simulink model "prs_agc"  (Simulink 8.7)
settings: Solver=ode45  StartTime=0.0  StopTime=100  RelTol=1e-3
values from neighbouring files (symbols this model uses):
  kd = GlobalBest.Position(3)    [prs_PSO.m]
  ki = GlobalBest.Position(2)    [prs_PSO.m]
  kp = GlobalBest.Position(1)    [prs_PSO.m]
libraries: simulink x2
settings Model: Creator=Prasun-EE  LastModifiedBy=User
settings DebuggingCC: UnderspecifiedInitializationDetection=Simplified  MergeDetectMultiDrivingBlocksExec=error
settings ConfigComp: CovSFcnEnable=off

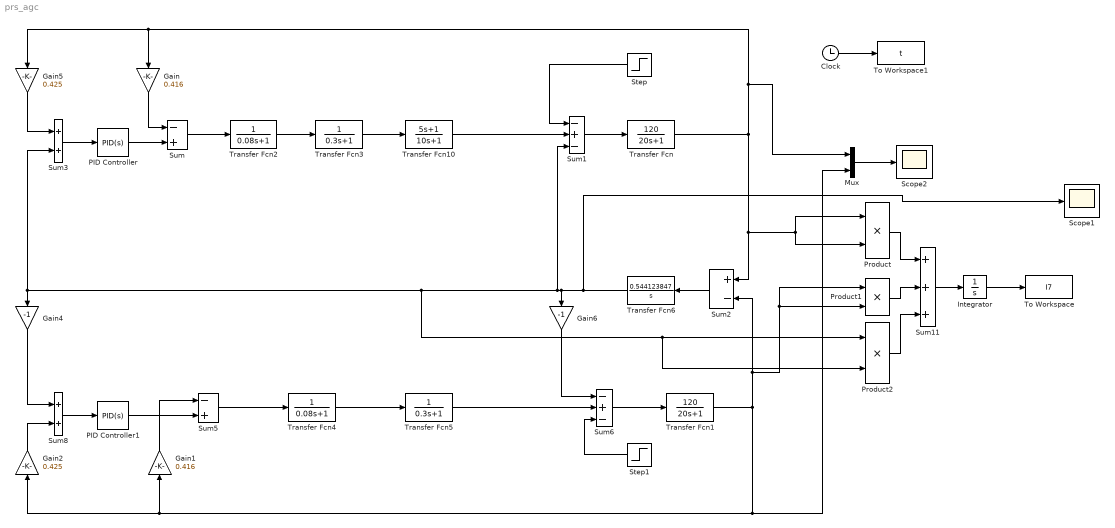
== system prs_agc ==
  Clock : Clock
  Gain : Gain  Gain=0.416
  Gain1 : Gain  Gain=0.416
  Gain2 : Gain  Gain=0.425
  Gain4 : Gain  Gain=-1
  Gain5 : Gain  Gain=0.425
  Gain6 : Gain  Gain=-1
  Integrator : Integrator  ZeroCross=off
  Mux : Mux  Inputs=2
  PID Controller : simulink/Continuous/PID Controller  Controller=PID  TimeDomain=Continuous-time  SampleTime=-1  IntegratorMethod=Forward Euler  FilterMethod=Forward Euler  Form=Parallel  UseFilter=on  ControllerParametersSource=internal  P=-kp  I=-ki  D=-kd  N=100  InitialConditionSource=internal  InitialConditionForIntegrator=0  InitialConditionForFilter=0  ExternalReset=none  LimitOutput=off  UpperSaturationLimit=inf  LowerSaturationLimit=-inf  LinearizeAsGain=on  AntiWindupMode=none  Kb=1  TrackingMode=off  Kt=1  PParamMin=[]  PParamMax=[]  IParamMin=[]  IParamMax=[]  DParamMin=[]  DParamMax=[]  NParamMin=[]  NParamMax=[]  KbParamMin=[]  KbParamMax=[]  KtParamMin=[]  KtParamMax=[]  POutMin=[]  POutMax=[]  IOutMin=[]  IOutMax=[]  DOutMin=[]  DOutMax=[]  NOutMin=[]  NOutMax=[]  KbOutMin=[]  KbOutMax=[]  KtOutMin=[]  KtOutMax=[]  IntegratorOutMin=[]  IntegratorOutMax=[]  FilterOutMin=[]  FilterOutMax=[]  SumOutMin=[]  SumOutMax=[]  SumI1OutMin=[]  SumI1OutMax=[]  SumI2OutMin=[]  SumI2OutMax=[]  SumI3OutMin=[]  SumI3OutMax=[]  SumDOutMin=[]  SumDOutMax=[]  SaturationOutMin=[]  SaturationOutMax=[]  IntegratorContinuousStateAttributes=''  IntegratorStateMustResolveToSignalObject=off  IntegratorRTWStateStorageClass=Auto  FilterContinuousStateAttributes=''  FilterStateMustResolveToSignalObject=off  FilterRTWStateStorageClass=Auto  DifferentiatorICPrevScaledInput=0  DifferentiatorOutMin=[]  DifferentiatorOutMax=[]
  PID Controller1 : simulink/Continuous/PID Controller  Controller=PID  TimeDomain=Continuous-time  SampleTime=-1  IntegratorMethod=Forward Euler  FilterMethod=Forward Euler  Form=Parallel  UseFilter=on  ControllerParametersSource=internal  P=-kp  I=-ki  D=-kd  N=100  InitialConditionSource=internal  InitialConditionForIntegrator=0  InitialConditionForFilter=0  ExternalReset=none  LimitOutput=off  UpperSaturationLimit=inf  LowerSaturationLimit=-inf  LinearizeAsGain=on  AntiWindupMode=none  Kb=1  TrackingMode=off  Kt=1  PParamMin=[]  PParamMax=[]  IParamMin=[]  IParamMax=[]  DParamMin=[]  DParamMax=[]  NParamMin=[]  NParamMax=[]  KbParamMin=[]  KbParamMax=[]  KtParamMin=[]  KtParamMax=[]  POutMin=[]  POutMax=[]  IOutMin=[]  IOutMax=[]  DOutMin=[]  DOutMax=[]  NOutMin=[]  NOutMax=[]  KbOutMin=[]  KbOutMax=[]  KtOutMin=[]  KtOutMax=[]  IntegratorOutMin=[]  IntegratorOutMax=[]  FilterOutMin=[]  FilterOutMax=[]  SumOutMin=[]  SumOutMax=[]  SumI1OutMin=[]  SumI1OutMax=[]  SumI2OutMin=[]  SumI2OutMax=[]  SumI3OutMin=[]  SumI3OutMax=[]  SumDOutMin=[]  SumDOutMax=[]  SaturationOutMin=[]  SaturationOutMax=[]  IntegratorContinuousStateAttributes=''  IntegratorStateMustResolveToSignalObject=off  IntegratorRTWStateStorageClass=Auto  FilterContinuousStateAttributes=''  FilterStateMustResolveToSignalObject=off  FilterRTWStateStorageClass=Auto  DifferentiatorICPrevScaledInput=0  DifferentiatorOutMin=[]  DifferentiatorOutMax=[]
  Product : Product  RndMeth=Zero
  Product1 : Product  RndMeth=Zero
  Product2 : Product  RndMeth=Zero
  Scope1 : Scope
  Scope2 : Scope
  Step : Step  Time=0  After=0.01  SampleTime=0
  Step1 : Step  Time=0  After=0  SampleTime=0
  Sum : Sum  Inputs=-+
  Sum1 : Sum  Inputs=-+-
  Sum11 : Sum  Inputs=+++
  Sum2 : Sum  Inputs=+-
  Sum3 : Sum
  Sum5 : Sum  Inputs=-+
  Sum6 : Sum  Inputs=-+-
  Sum8 : Sum
  To Workspace : ToWorkspace  VariableName=I7  SampleTime=-1
  To Workspace1 : ToWorkspace  VariableName=t  SampleTime=-1
  Transfer Fcn : TransferFcn  Numerator=[120]  Denominator=[20 1]
  Transfer Fcn1 : TransferFcn  Numerator=[120]  Denominator=[20 1]
  Transfer Fcn10 : TransferFcn  Numerator=[5 1]  Denominator=[10 1]
  Transfer Fcn2 : TransferFcn  Denominator=[0.08 1]
  Transfer Fcn3 : TransferFcn  Denominator=[0.3 1]
  Transfer Fcn4 : TransferFcn  Denominator=[0.08 1]
  Transfer Fcn5 : TransferFcn  Denominator=[0.3 1]
  Transfer Fcn6 : TransferFcn  Numerator=[0.544123847]  Denominator=[1 0]
  wires:
  Sum6/1 -> Transfer Fcn1/1
  Transfer Fcn1/1 -> Sum2/2, Product1/1, Product1/2, Gain1/1, Gain2/1, Mux/2
  Sum2/1 -> Transfer Fcn6/1
  Sum8/1 -> PID Controller1/1
  Gain2/1 -> Sum8/2
  Gain6/1 -> Sum6/1
  Gain4/1 -> Sum8/1
  Transfer Fcn6/1 -> Scope1/1, Gain6/1, Sum1/3, Sum3/2, Gain4/1, Product2/1, Product2/2
  Step1/1 -> Sum6/3
  Sum1/1 -> Transfer Fcn/1
  Transfer Fcn3/1 -> Transfer Fcn10/1
  Sum/1 -> Transfer Fcn2/1
  Transfer Fcn/1 -> Gain/1, Gain5/1, Mux/1, Sum2/1, Product/1, Product/2
  Transfer Fcn2/1 -> Transfer Fcn3/1
  Gain/1 -> Sum/1
  Gain5/1 -> Sum3/1
  Mux/1 -> Scope2/1
  Sum11/1 -> Integrator/1
  Product/1 -> Sum11/1
  Product1/1 -> Sum11/2
  Product2/1 -> Sum11/3
  Integrator/1 -> To Workspace/1
  Clock/1 -> To Workspace1/1
  Sum3/1 -> PID Controller/1
  Sum5/1 -> Transfer Fcn4/1
  Gain1/1 -> Sum5/1
  PID Controller1/1 -> Sum5/2
  Transfer Fcn4/1 -> Transfer Fcn5/1
  Step/1 -> Sum1/1
  PID Controller/1 -> Sum/2
  Transfer Fcn10/1 -> Sum1/2
  Transfer Fcn5/1 -> Sum6/2
